simulink model "gm_multi_module_phase_shift_generator_built_in_counter"  (R2025b)
settings: Solver=FixedStepDiscrete  StartTime=0.0  StopTime=10e3  RelTol=1e-3
libraries: hdlmdlgenlib x1
settings Model: Creator=KoayXianCong  LastModifiedBy=KoayXianCong
settings OptimizationCC: BlockReduction=off  ConditionallyExecuteInputs=off  DefaultParameterBehavior=Inlined  InheritOutputTypeSmallerThanSingle=on
settings DebuggingCC: ArtificialAlgebraicLoopMsg=error  InheritedTsInSrcMsg=none  SingleTaskRateTransMsg=error
settings HardwareCC: ProdBitPerPointer=32.0  ProdBitPerSizeT=32.0  ProdBitPerPtrDiffT=32.0  ProdLargestAtomicFloat=None  ProdIntDivRoundTo=Undefined  ProdEndianess=Unspecified  ProdWordSize=32.0  ProdHWDeviceType=ASIC/FPGA->ASIC/FPGA  TargetBitPerPointer=64.0  TargetBitPerSizeT=64.0  TargetBitPerPtrDiffT=64.0  TargetLongLongMode=on  TargetIntDivRoundTo=Zero  TargetEndianess=LittleEndian  TargetWordSize=64.0  TargetHWDeviceType=Custom Processor->MATLAB Host Computer  ProdEqTarget=off

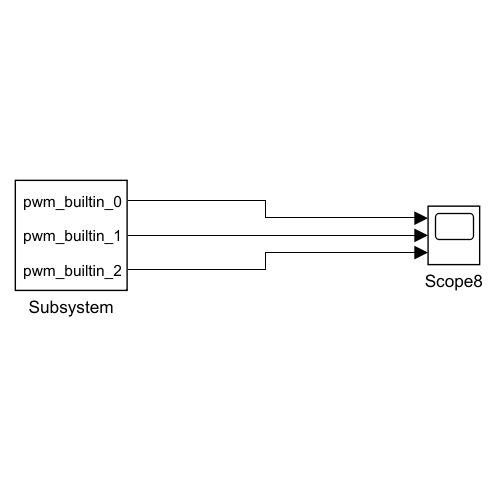
[thumbnail: Simulink's stored preview of the top-level diagram]
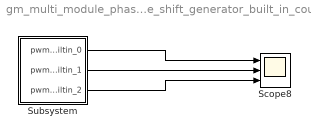
== system gm_multi_module_phase_shift_generator_built_in_counter ==
  Scope8 : Scope  NumInputPorts=3
      settings: ActiveDisplayYMinimum=-1  ActiveDisplayYMaximum=1  DataLoggingVariableName=ScopeData10  DataLoggingSaveFormat=Array
  Subsystem : Subsystem
  wires:
  Subsystem/3(pwm_builtin_2) -> Scope8/3
  Subsystem/2(pwm_builtin_1) -> Scope8/2
  Subsystem/1(pwm_builtin_0) -> Scope8/1

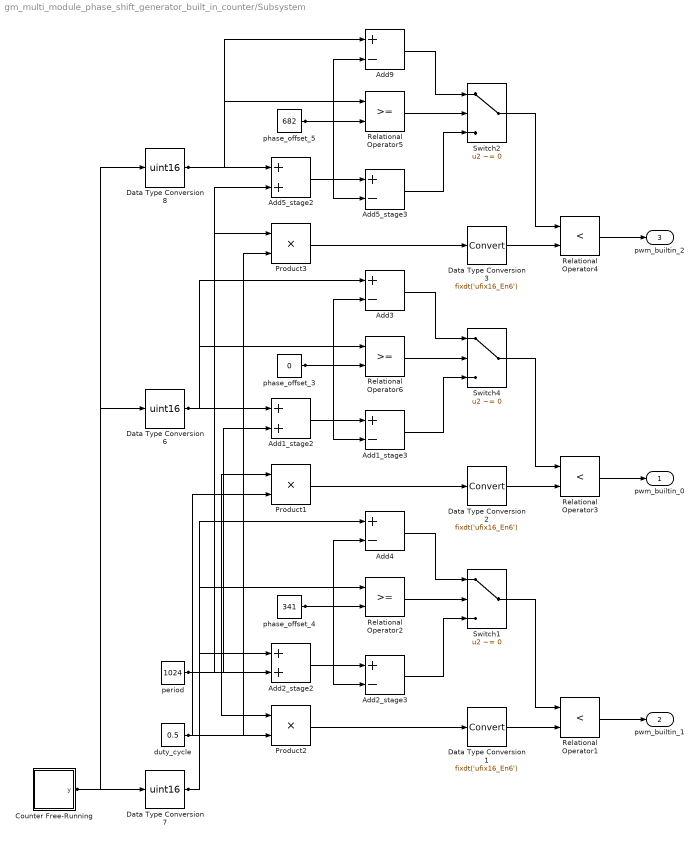
== system gm_multi_module_phase_shift_generator_built_in_counter/Subsystem ==
  Add1_stage2 : Sum  OutDataTypeStr=fixdt(0, 17, 0)  AccumDataTypeStr=fixdt(1, 23, 4)  SampleTime=1
  Add1_stage3 : Sum  Inputs=+-  OutDataTypeStr=fixdt(1, 23, 4)  AccumDataTypeStr=fixdt(1, 23, 4)  SampleTime=1
  Add2_stage2 : Sum  OutDataTypeStr=fixdt(0, 17, 0)  AccumDataTypeStr=fixdt(1, 25, 7)  SampleTime=1
  Add2_stage3 : Sum  Inputs=+-  OutDataTypeStr=fixdt(1, 25, 7)  AccumDataTypeStr=fixdt(1, 25, 7)  SampleTime=1
  Add3 : Sum  Inputs=+-  OutDataTypeStr=fixdt(1, 22, 4)  AccumDataTypeStr=fixdt(1, 22, 4)  SampleTime=1
  Add4 : Sum  Inputs=+-  OutDataTypeStr=fixdt(1, 24, 7)  AccumDataTypeStr=fixdt(1, 24, 7)  SampleTime=1
  Add5_stage2 : Sum  OutDataTypeStr=fixdt(0, 17, 0)  AccumDataTypeStr=fixdt(1, 24, 6)  SampleTime=1
  Add5_stage3 : Sum  Inputs=+-  OutDataTypeStr=fixdt(1, 24, 6)  AccumDataTypeStr=fixdt(1, 24, 6)  SampleTime=1
  Add9 : Sum  Inputs=+-  OutDataTypeStr=fixdt(1, 23, 6)  AccumDataTypeStr=fixdt(1, 23, 6)  SampleTime=1
  Counter Free-Running : Subsystem  mask(Counter Free-Running){NumBits=double(10), tsamp=double(1)}
      mask prompts: NumBits "Simulink:masks:NumberOfBits_MP"; tsamp "Simulink:masks:SampleTime_MP"
      mask help: Simulink:masks:CounterFreeRunning_MD
  Data Type Conversion1 : DataTypeConversion  OutDataTypeStr=fixdt('ufix16_En6')
  Data Type Conversion2 : DataTypeConversion  OutDataTypeStr=fixdt('ufix16_En6')
  Data Type Conversion3 : DataTypeConversion  OutDataTypeStr=fixdt('ufix16_En6')
  Data Type Conversion6 : DataTypeConversion  OutDataTypeStr=uint16  SampleTime=1  SaturateOnIntegerOverflow=off  RndMeth=Floor
  Data Type Conversion7 : DataTypeConversion  OutDataTypeStr=uint16  SampleTime=1  SaturateOnIntegerOverflow=off  RndMeth=Floor
  Data Type Conversion8 : DataTypeConversion  OutDataTypeStr=uint16  SampleTime=1  SaturateOnIntegerOverflow=off  RndMeth=Floor
  Product1 : Product  Inputs=**  OutDataTypeStr=fixdt(0, 16, 6)  SampleTime=1
  Product2 : Product  Inputs=**  OutDataTypeStr=fixdt(0, 16, 6)  SampleTime=1
  Product3 : Product  Inputs=**  OutDataTypeStr=fixdt(0, 16, 6)  SampleTime=1
  Relational Operator1 : RelationalOperator  Operator=<  OutDataTypeStr=boolean  SampleTime=1  InputSameDT=off
  Relational Operator2 : RelationalOperator  OutDataTypeStr=boolean  SampleTime=1  InputSameDT=off
  Relational Operator3 : RelationalOperator  Operator=<  OutDataTypeStr=boolean  SampleTime=1  InputSameDT=off
  Relational Operator4 : RelationalOperator  Operator=<  OutDataTypeStr=boolean  SampleTime=1  InputSameDT=off
  Relational Operator5 : RelationalOperator  OutDataTypeStr=boolean  SampleTime=1  InputSameDT=off
  Relational Operator6 : RelationalOperator  OutDataTypeStr=boolean  SampleTime=1  InputSameDT=off
  Switch1 : Switch  Criteria=u2 ~= 0  Threshold="fi(0,0,1,0,\"hex\",\"0\")"  OutDataTypeStr=fixdt(1, 25, 7)  SampleTime=1  SaturateOnIntegerOverflow=off  InputSameDT=off
  Switch2 : Switch  Criteria=u2 ~= 0  Threshold="fi(0,0,1,0,\"hex\",\"0\")"  OutDataTypeStr=fixdt(1, 24, 6)  SampleTime=1  SaturateOnIntegerOverflow=off  InputSameDT=off
  Switch4 : Switch  Criteria=u2 ~= 0  Threshold="fi(0,0,1,0,\"hex\",\"0\")"  OutDataTypeStr=fixdt(1, 23, 4)  SampleTime=1  SaturateOnIntegerOverflow=off  InputSameDT=off
  duty_cycle : Constant  Value=0.5  OutDataTypeStr=fixdt(0, 16, 16)  SampleTime=1
  period : Constant  Value=1024  OutDataTypeStr=uint16  SampleTime=1
  phase_offset_3 : Constant  Value=0  OutDataTypeStr=fixdt(1, 16, 4)  SampleTime=1
  phase_offset_4 : Constant  Value=341  OutDataTypeStr=fixdt(0, 16, 7)  SampleTime=1
  phase_offset_5 : Constant  Value=682  OutDataTypeStr=fixdt(0, 16, 6)  SampleTime=1
  pwm_builtin_0 : Outport  SampleTime=1
  pwm_builtin_1 : Outport  Port=2  SampleTime=1
  pwm_builtin_2 : Outport  Port=3  SampleTime=1
  wires:
  Data Type Conversion3/1 -> Relational Operator4/2
  phase_offset_4/1 -> Relational Operator2/2, Add4/2, Add2_stage3/2
  Counter Free-Running/1(y) -> Data Type Conversion8/1, Data Type Conversion7/1, Data Type Conversion6/1
  Data Type Conversion8/1 -> Add9/1, Relational Operator5/1, Add5_stage2/1
  Data Type Conversion6/1 -> Add3/1, Add1_stage2/1, Relational Operator6/1
  phase_offset_5/1 -> Relational Operator5/2, Add9/2, Add5_stage3/2
  period/1 -> Add5_stage2/2, Add1_stage2/2, Product3/1, Product2/1, Product1/1, Add2_stage2/2
  Product1/1 -> Data Type Conversion2/1
  duty_cycle/1 -> Product2/2, Product3/2, Product1/2
  Data Type Conversion7/1 -> Relational Operator2/1, Add2_stage2/1, Add4/1
  Add5_stage2/1 -> Add5_stage3/1
  Product3/1 -> Data Type Conversion3/1
  phase_offset_3/1 -> Relational Operator6/2, Add3/2, Add1_stage3/2
  Switch1/1 -> Relational Operator1/1
  Add1_stage2/1 -> Add1_stage3/1
  Add2_stage2/1 -> Add2_stage3/1
  Product2/1 -> Data Type Conversion1/1
  Add9/1 -> Switch2/1
  Relational Operator5/1 -> Switch2/2
  Add5_stage3/1 -> Switch2/3
  Add3/1 -> Switch4/1
  Relational Operator6/1 -> Switch4/2
  Add1_stage3/1 -> Switch4/3
  Add4/1 -> Switch1/1
  Relational Operator2/1 -> Switch1/2
  Add2_stage3/1 -> Switch1/3
  Switch2/1 -> Relational Operator4/1
  Switch4/1 -> Relational Operator3/1
  Data Type Conversion2/1 -> Relational Operator3/2
  Data Type Conversion1/1 -> Relational Operator1/2
  Relational Operator4/1 -> pwm_builtin_2/1
  Relational Operator3/1 -> pwm_builtin_0/1
  Relational Operator1/1 -> pwm_builtin_1/1

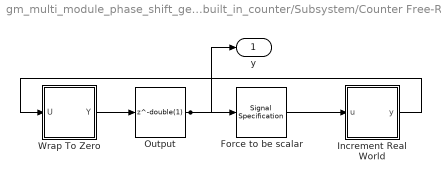
== system gm_multi_module_phase_shift_generator_built_in_counter/Subsystem/Counter Free-Running ==
  Force to be scalar : SignalSpecification  OutDataTypeStr=fixdt(0, 10, 0)  Dimensions=1
  Increment Real World : Subsystem  mask(Real World Value Increment){}
      mask help: Simulink:masks:RealWorldValueIncrement_MD
      mask Display: disp('V++')
  Output : Delay  DelayLength=double(1)  InitialCondition=0  SampleTime=1
  Wrap To Zero : Subsystem  mask(Wrap To Zero){Threshold=double(1023)}
      mask prompts: Threshold "Simulink:masks:Threshold_MP"
      mask help: Simulink:masks:WrapToZero_MD
  y : Outport  SampleTime=1
  wires:
  Wrap To Zero/1(Y) -> Output/1
  Output/1 -> Force to be scalar/1, y/1
  Force to be scalar/1 -> Increment Real World/1(u)
  Increment Real World/1(y) -> Wrap To Zero/1(U)

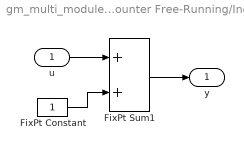
== system gm_multi_module_phase_shift_generator_built_in_counter/Subsystem/Counter Free-Running/Increment Real World ==
  u : Inport  OutDataTypeStr=fixdt(0, 10, 0)  SampleTime=1
  FixPt Constant : Constant  DisableCoverage=on  OutDataTypeStr=fixdt(0, 10, 0)  SampleTime=-1
  FixPt Sum1 : Sum  OutDataTypeStr=fixdt(0, 10, 0)  InputSameDT=on  LockScale=on
  y : Outport  SampleTime=1
  wires:
  u/1 -> FixPt Sum1/1
  FixPt Constant/1 -> FixPt Sum1/2
  FixPt Sum1/1 -> y/1

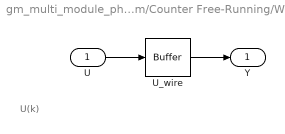
== system gm_multi_module_phase_shift_generator_built_in_counter/Subsystem/Counter Free-Running/Wrap To Zero ==
  note: U(k)
  U : Inport  OutDataTypeStr=fixdt(0, 10, 0)  SampleTime=1
  U_wire : hdlmdlgenlib/Buffer
  Y : Outport  SampleTime=1  InitialOutput=0
  wires:
  U/1 -> U_wire/1
  U_wire/1 -> Y/1
